simulink model "PhysicalLeanBroth"  (R2026a)
settings: Solver=VariableStepAuto  StopTime=14400
undefined symbols (not defined in the file or in its folder): Fault_T_Kettle1, Fault_T_Kettle2, Fault_T_Pack, Fault_T_Prep, Fault_T_QC, LB_PackRate_bph, LB_QCRate_bph, LB_Resupply_bph, Recipe_Block_s, Recipe_Count, Resupply_Cutoff_T, Transport_Latency_s, Transport_Rate_bph
settings Model: DataDictionary=PhysicalLeanBrothData.sldd  Creator=sarah  LastModifiedBy=sarah

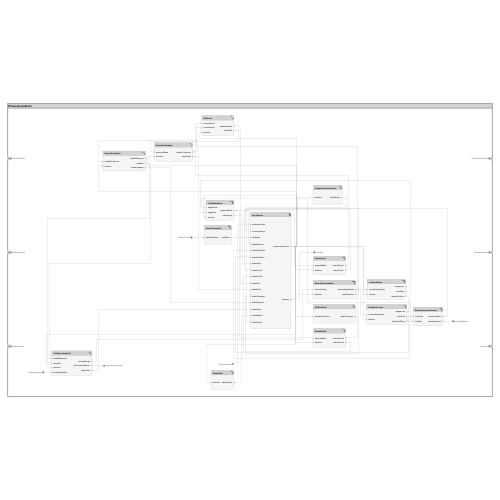
[thumbnail: Simulink's stored preview of the top-level diagram]
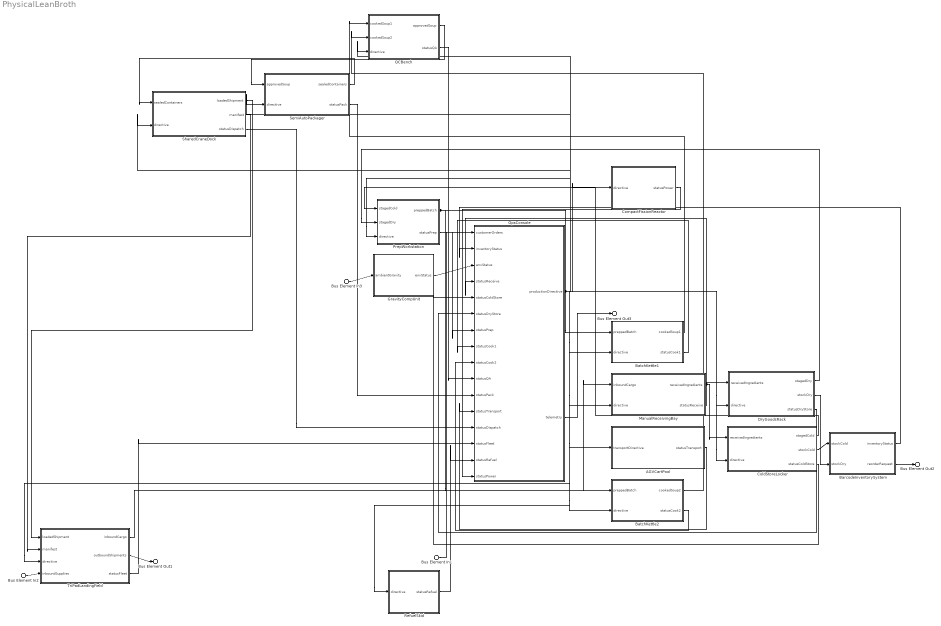
== system PhysicalLeanBroth ==
  Bus Element In1 : Inport  PortName=CustomerOrders
  Bus Element In2 : Inport  Port=2  PortName=InboundSupplies
  Bus Element In3 : Inport  Port=3  PortName=AmbientGravity
  AGVCartPool : Subsystem
      settings: PortSchema="{\"entries\":[{\"content\":{\"headerSize\":26,\"margin\":15,\"minimumSpacing\":25,\"sides\":[{\"content\":{\"connectorIds\":[\"In1\"]},\"type\":\"ConnectorPlacement.EquallySpacedRectSide\",\"uuid\":\"f830f98a-8e8b-4468-adf4-d6eab644987f\"},{\"content\":{\"connectorIds\":[\"Out1\"],\"side\":\"RIGHT\"},\"type\":\"ConnectorPlacement.EquallySpacedRectSide\",\"uuid\":\"7e0d0116-b3ba-4668-b638-30d0f54ba087\"},{\"content\":{\"side\":\"TOP\"},\"type\":\"ConnectorPlacement.EquallySpacedRectSide\",\"uuid\":\"7b4146d3-46d2-45ca-8c34-b106f0d8cedd\"}]},\"type\":\"ConnectorPlacement.EquallySpacedConnector\",\"uuid\":\"3d911b2d-a78f-42ea-b869-5e09982d9f54\"}],\"packageUris\":[\"http://schema.mathworks.com/mf0/Connector/R2020b\"],\"version\":\"1.0\"}"
  BarcodeInventorySystem : Subsystem
      settings: PortSchema="{\"entries\":[{\"content\":{\"headerSize\":26,\"margin\":15,\"minimumSpacing\":25,\"sides\":[{\"content\":{\"connectorIds\":[\"In1\",\"In2\"]},\"type\":\"ConnectorPlacement.EquallySpacedRectSide\",\"uuid\":\"f830f98a-8e8b-4468-adf4-d6eab644987f\"},{\"content\":{\"connectorIds\":[\"Out1\",\"Out2\"],\"side\":\"RIGHT\"},\"type\":\"ConnectorPlacement.EquallySpacedRectSide\",\"uuid\":\"7e0d0116-b3ba-4668-b638-30d0f54ba087\"},{\"content\":{\"side\":\"TOP\"},\"type\":\"ConnectorPlacement.EquallySpacedRectSide\",\"uuid\":\"7b4146d3-46d2-45ca-8c34-b106f0d8cedd\"}]},\"type\":\"ConnectorPlacement.EquallySpacedConnector\",\"uuid\":\"3d911b2d-a78f-42ea-b869-5e09982d9f54\"}],\"packageUris\":[\"http://schema.mathworks.com/mf0/Connector/R2020b\"],\"version\":\"1.0\"}"
  BatchKettle1 : Subsystem
      settings: PortSchema="{\"entries\":[{\"content\":{\"headerSize\":26,\"margin\":15,\"minimumSpacing\":25,\"sides\":[{\"content\":{\"connectorIds\":[\"In1\",\"In2\"]},\"type\":\"ConnectorPlacement.EquallySpacedRectSide\",\"uuid\":\"f830f98a-8e8b-4468-adf4-d6eab644987f\"},{\"content\":{\"connectorIds\":[\"Out1\",\"Out2\"],\"side\":\"RIGHT\"},\"type\":\"ConnectorPlacement.EquallySpacedRectSide\",\"uuid\":\"7e0d0116-b3ba-4668-b638-30d0f54ba087\"},{\"content\":{\"side\":\"TOP\"},\"type\":\"ConnectorPlacement.EquallySpacedRectSide\",\"uuid\":\"7b4146d3-46d2-45ca-8c34-b106f0d8cedd\"}]},\"type\":\"ConnectorPlacement.EquallySpacedConnector\",\"uuid\":\"3d911b2d-a78f-42ea-b869-5e09982d9f54\"}],\"packageUris\":[\"http://schema.mathworks.com/mf0/Connector/R2020b\"],\"version\":\"1.0\"}"
  BatchKettle2 : Subsystem
      settings: PortSchema="{\"entries\":[{\"content\":{\"headerSize\":26,\"margin\":15,\"minimumSpacing\":25,\"sides\":[{\"content\":{\"connectorIds\":[\"In1\",\"In2\"]},\"type\":\"ConnectorPlacement.EquallySpacedRectSide\",\"uuid\":\"f830f98a-8e8b-4468-adf4-d6eab644987f\"},{\"content\":{\"connectorIds\":[\"Out1\",\"Out2\"],\"side\":\"RIGHT\"},\"type\":\"ConnectorPlacement.EquallySpacedRectSide\",\"uuid\":\"7e0d0116-b3ba-4668-b638-30d0f54ba087\"},{\"content\":{\"side\":\"TOP\"},\"type\":\"ConnectorPlacement.EquallySpacedRectSide\",\"uuid\":\"7b4146d3-46d2-45ca-8c34-b106f0d8cedd\"}]},\"type\":\"ConnectorPlacement.EquallySpacedConnector\",\"uuid\":\"3d911b2d-a78f-42ea-b869-5e09982d9f54\"}],\"packageUris\":[\"http://schema.mathworks.com/mf0/Connector/R2020b\"],\"version\":\"1.0\"}"
  ColdStoreLocker : Subsystem
      settings: PortSchema="{\"entries\":[{\"content\":{\"headerSize\":26,\"margin\":15,\"minimumSpacing\":25,\"sides\":[{\"content\":{\"connectorIds\":[\"In1\",\"In2\"]},\"type\":\"ConnectorPlacement.EquallySpacedRectSide\",\"uuid\":\"f830f98a-8e8b-4468-adf4-d6eab644987f\"},{\"content\":{\"connectorIds\":[\"Out1\",\"Out2\",\"Out3\"],\"side\":\"RIGHT\"},\"type\":\"ConnectorPlacement.EquallySpacedRectSide\",\"uuid\":\"7e0d0116-b3ba-4668-b638-30d0f54ba087\"},{\"content\":{\"side\":\"TOP\"},\"type\":\"ConnectorPlacement.EquallySpacedRectSide\",\"uuid\":\"7b4146d3-46d2-45ca-8c34-b106f0d8cedd\"}]},\"type\":\"ConnectorPlacement.EquallySpacedConnector\",\"uuid\":\"3d911b2d-a78f-42ea-b869-5e09982d9f54\"}],\"packageUris\":[\"http://schema.mathworks.com/mf0/Connector/R2020b\"],\"version\":\"1.0\"}"
  CompactFissionReactor : Subsystem
      settings: PortSchema="{\"entries\":[{\"content\":{\"headerSize\":26,\"margin\":15,\"minimumSpacing\":25,\"sides\":[{\"content\":{\"connectorIds\":[\"In1\"]},\"type\":\"ConnectorPlacement.EquallySpacedRectSide\",\"uuid\":\"f830f98a-8e8b-4468-adf4-d6eab644987f\"},{\"content\":{\"connectorIds\":[\"Out1\"],\"side\":\"RIGHT\"},\"type\":\"ConnectorPlacement.EquallySpacedRectSide\",\"uuid\":\"7e0d0116-b3ba-4668-b638-30d0f54ba087\"},{\"content\":{\"side\":\"TOP\"},\"type\":\"ConnectorPlacement.EquallySpacedRectSide\",\"uuid\":\"7b4146d3-46d2-45ca-8c34-b106f0d8cedd\"}]},\"type\":\"ConnectorPlacement.EquallySpacedConnector\",\"uuid\":\"3d911b2d-a78f-42ea-b869-5e09982d9f54\"}],\"packageUris\":[\"http://schema.mathworks.com/mf0/Connector/R2020b\"],\"version\":\"1.0\"}"
  DryGoodsRack : Subsystem
      settings: PortSchema="{\"entries\":[{\"content\":{\"headerSize\":26,\"margin\":15,\"minimumSpacing\":25,\"sides\":[{\"content\":{\"connectorIds\":[\"In1\",\"In2\"]},\"type\":\"ConnectorPlacement.EquallySpacedRectSide\",\"uuid\":\"f830f98a-8e8b-4468-adf4-d6eab644987f\"},{\"content\":{\"connectorIds\":[\"Out1\",\"Out2\",\"Out3\"],\"side\":\"RIGHT\"},\"type\":\"ConnectorPlacement.EquallySpacedRectSide\",\"uuid\":\"7e0d0116-b3ba-4668-b638-30d0f54ba087\"},{\"content\":{\"side\":\"TOP\"},\"type\":\"ConnectorPlacement.EquallySpacedRectSide\",\"uuid\":\"7b4146d3-46d2-45ca-8c34-b106f0d8cedd\"}]},\"type\":\"ConnectorPlacement.EquallySpacedConnector\",\"uuid\":\"3d911b2d-a78f-42ea-b869-5e09982d9f54\"}],\"packageUris\":[\"http://schema.mathworks.com/mf0/Connector/R2020b\"],\"version\":\"1.0\"}"
  GravityCompUnit : Subsystem
      settings: PortSchema="{\"entries\":[{\"content\":{\"headerSize\":26,\"margin\":15,\"minimumSpacing\":25,\"sides\":[{\"content\":{\"connectorIds\":[\"In1\"]},\"type\":\"ConnectorPlacement.EquallySpacedRectSide\",\"uuid\":\"f830f98a-8e8b-4468-adf4-d6eab644987f\"},{\"content\":{\"connectorIds\":[\"Out1\"],\"side\":\"RIGHT\"},\"type\":\"ConnectorPlacement.EquallySpacedRectSide\",\"uuid\":\"7e0d0116-b3ba-4668-b638-30d0f54ba087\"},{\"content\":{\"side\":\"TOP\"},\"type\":\"ConnectorPlacement.EquallySpacedRectSide\",\"uuid\":\"7b4146d3-46d2-45ca-8c34-b106f0d8cedd\"}]},\"type\":\"ConnectorPlacement.EquallySpacedConnector\",\"uuid\":\"3d911b2d-a78f-42ea-b869-5e09982d9f54\"}],\"packageUris\":[\"http://schema.mathworks.com/mf0/Connector/R2020b\"],\"version\":\"1.0\"}"
  ManualReceivingBay : Subsystem
      settings: PortSchema="{\"entries\":[{\"content\":{\"headerSize\":26,\"margin\":15,\"minimumSpacing\":25,\"sides\":[{\"content\":{\"connectorIds\":[\"In1\",\"In2\"]},\"type\":\"ConnectorPlacement.EquallySpacedRectSide\",\"uuid\":\"f830f98a-8e8b-4468-adf4-d6eab644987f\"},{\"content\":{\"connectorIds\":[\"Out1\",\"Out2\"],\"side\":\"RIGHT\"},\"type\":\"ConnectorPlacement.EquallySpacedRectSide\",\"uuid\":\"7e0d0116-b3ba-4668-b638-30d0f54ba087\"},{\"content\":{\"side\":\"TOP\"},\"type\":\"ConnectorPlacement.EquallySpacedRectSide\",\"uuid\":\"7b4146d3-46d2-45ca-8c34-b106f0d8cedd\"}]},\"type\":\"ConnectorPlacement.EquallySpacedConnector\",\"uuid\":\"3d911b2d-a78f-42ea-b869-5e09982d9f54\"}],\"packageUris\":[\"http://schema.mathworks.com/mf0/Connector/R2020b\"],\"version\":\"1.0\"}"
  OpsConsole : Subsystem
      settings: PortSchema="{\"entries\":[{\"content\":{\"headerSize\":26,\"margin\":15,\"minimumSpacing\":25,\"sides\":[{\"content\":{\"connectorIds\":[\"In1\",\"In2\",\"In3\",\"In4\",\"In5\",\"In6\",\"In7\",\"In8\",\"In9\",\"In10\",\"In11\",\"In12\",\"In13\",\"In14\",\"In15\",\"In16\"]},\"type\":\"ConnectorPlacement.EquallySpacedRectSide\",\"uuid\":\"f830f98a-8e8b-4468-adf4-d6eab644987f\"},{\"content\":{\"connectorIds\":[\"Out1\",\"Out2\"],\"side\":\"RIGHT\"},\"type\":\"ConnectorPlacement.EquallySpacedRectSide\",\"uuid\":\"7e0d0116-b3ba-4668-b638-30d0f54ba087\"},{\"content\":{\"side\":\"TOP\"},\"type\":\"ConnectorPlacement.EquallySpacedRectSide\",\"uuid\":\"7b4146d3-46d2-45ca-8c34-b106f0d8cedd\"}]},\"type\":\"ConnectorPlacement.EquallySpacedConnector\",\"uuid\":\"3d911b2d-a78f-42ea-b869-5e09982d9f54\"}],\"packageUris\":[\"http://schema.mathworks.com/mf0/Connector/R2020b\"],\"version\":\"1.0\"}"
  PrepWorkstation : Subsystem
      settings: PortSchema="{\"entries\":[{\"content\":{\"headerSize\":26,\"margin\":15,\"minimumSpacing\":25,\"sides\":[{\"content\":{\"connectorIds\":[\"In1\",\"In2\",\"In3\"]},\"type\":\"ConnectorPlacement.EquallySpacedRectSide\",\"uuid\":\"f830f98a-8e8b-4468-adf4-d6eab644987f\"},{\"content\":{\"connectorIds\":[\"Out1\",\"Out2\"],\"side\":\"RIGHT\"},\"type\":\"ConnectorPlacement.EquallySpacedRectSide\",\"uuid\":\"7e0d0116-b3ba-4668-b638-30d0f54ba087\"},{\"content\":{\"side\":\"TOP\"},\"type\":\"ConnectorPlacement.EquallySpacedRectSide\",\"uuid\":\"7b4146d3-46d2-45ca-8c34-b106f0d8cedd\"}]},\"type\":\"ConnectorPlacement.EquallySpacedConnector\",\"uuid\":\"3d911b2d-a78f-42ea-b869-5e09982d9f54\"}],\"packageUris\":[\"http://schema.mathworks.com/mf0/Connector/R2020b\"],\"version\":\"1.0\"}"
  QCBench : Subsystem
      settings: PortSchema="{\"entries\":[{\"content\":{\"headerSize\":26,\"margin\":15,\"minimumSpacing\":25,\"sides\":[{\"content\":{\"connectorIds\":[\"In1\",\"In2\",\"In3\"]},\"type\":\"ConnectorPlacement.EquallySpacedRectSide\",\"uuid\":\"f830f98a-8e8b-4468-adf4-d6eab644987f\"},{\"content\":{\"connectorIds\":[\"Out1\",\"Out2\"],\"side\":\"RIGHT\"},\"type\":\"ConnectorPlacement.EquallySpacedRectSide\",\"uuid\":\"7e0d0116-b3ba-4668-b638-30d0f54ba087\"},{\"content\":{\"side\":\"TOP\"},\"type\":\"ConnectorPlacement.EquallySpacedRectSide\",\"uuid\":\"7b4146d3-46d2-45ca-8c34-b106f0d8cedd\"}]},\"type\":\"ConnectorPlacement.EquallySpacedConnector\",\"uuid\":\"3d911b2d-a78f-42ea-b869-5e09982d9f54\"}],\"packageUris\":[\"http://schema.mathworks.com/mf0/Connector/R2020b\"],\"version\":\"1.0\"}"
  RefuelSkid : Subsystem
      settings: PortSchema="{\"entries\":[{\"content\":{\"headerSize\":26,\"margin\":15,\"minimumSpacing\":25,\"sides\":[{\"content\":{\"connectorIds\":[\"In1\"]},\"type\":\"ConnectorPlacement.EquallySpacedRectSide\",\"uuid\":\"f830f98a-8e8b-4468-adf4-d6eab644987f\"},{\"content\":{\"connectorIds\":[\"Out1\"],\"side\":\"RIGHT\"},\"type\":\"ConnectorPlacement.EquallySpacedRectSide\",\"uuid\":\"7e0d0116-b3ba-4668-b638-30d0f54ba087\"},{\"content\":{\"side\":\"TOP\"},\"type\":\"ConnectorPlacement.EquallySpacedRectSide\",\"uuid\":\"7b4146d3-46d2-45ca-8c34-b106f0d8cedd\"}]},\"type\":\"ConnectorPlacement.EquallySpacedConnector\",\"uuid\":\"3d911b2d-a78f-42ea-b869-5e09982d9f54\"}],\"packageUris\":[\"http://schema.mathworks.com/mf0/Connector/R2020b\"],\"version\":\"1.0\"}"
  SemiAutoPackager : Subsystem
      settings: PortSchema="{\"entries\":[{\"content\":{\"headerSize\":26,\"margin\":15,\"minimumSpacing\":25,\"sides\":[{\"content\":{\"connectorIds\":[\"In1\",\"In2\"]},\"type\":\"ConnectorPlacement.EquallySpacedRectSide\",\"uuid\":\"f830f98a-8e8b-4468-adf4-d6eab644987f\"},{\"content\":{\"connectorIds\":[\"Out1\",\"Out2\"],\"side\":\"RIGHT\"},\"type\":\"ConnectorPlacement.EquallySpacedRectSide\",\"uuid\":\"7e0d0116-b3ba-4668-b638-30d0f54ba087\"},{\"content\":{\"side\":\"TOP\"},\"type\":\"ConnectorPlacement.EquallySpacedRectSide\",\"uuid\":\"7b4146d3-46d2-45ca-8c34-b106f0d8cedd\"}]},\"type\":\"ConnectorPlacement.EquallySpacedConnector\",\"uuid\":\"3d911b2d-a78f-42ea-b869-5e09982d9f54\"}],\"packageUris\":[\"http://schema.mathworks.com/mf0/Connector/R2020b\"],\"version\":\"1.0\"}"
  SharedCraneDock : Subsystem
      settings: PortSchema="{\"entries\":[{\"content\":{\"headerSize\":26,\"margin\":15,\"minimumSpacing\":25,\"sides\":[{\"content\":{\"connectorIds\":[\"In1\",\"In2\"]},\"type\":\"ConnectorPlacement.EquallySpacedRectSide\",\"uuid\":\"f830f98a-8e8b-4468-adf4-d6eab644987f\"},{\"content\":{\"connectorIds\":[\"Out1\",\"Out2\",\"Out3\"],\"side\":\"RIGHT\"},\"type\":\"ConnectorPlacement.EquallySpacedRectSide\",\"uuid\":\"7e0d0116-b3ba-4668-b638-30d0f54ba087\"},{\"content\":{\"side\":\"TOP\"},\"type\":\"ConnectorPlacement.EquallySpacedRectSide\",\"uuid\":\"7b4146d3-46d2-45ca-8c34-b106f0d8cedd\"}]},\"type\":\"ConnectorPlacement.EquallySpacedConnector\",\"uuid\":\"3d911b2d-a78f-42ea-b869-5e09982d9f54\"}],\"packageUris\":[\"http://schema.mathworks.com/mf0/Connector/R2020b\"],\"version\":\"1.0\"}"
  TriPadLandingField : Subsystem
      settings: PortSchema="{\"entries\":[{\"content\":{\"headerSize\":26,\"margin\":15,\"minimumSpacing\":25,\"sides\":[{\"content\":{\"connectorIds\":[\"In1\",\"In2\",\"In3\",\"In4\"]},\"type\":\"ConnectorPlacement.EquallySpacedRectSide\",\"uuid\":\"f830f98a-8e8b-4468-adf4-d6eab644987f\"},{\"content\":{\"connectorIds\":[\"Out1\",\"Out2\",\"Out3\"],\"side\":\"RIGHT\"},\"type\":\"ConnectorPlacement.EquallySpacedRectSide\",\"uuid\":\"7e0d0116-b3ba-4668-b638-30d0f54ba087\"},{\"content\":{\"side\":\"TOP\"},\"type\":\"ConnectorPlacement.EquallySpacedRectSide\",\"uuid\":\"7b4146d3-46d2-45ca-8c34-b106f0d8cedd\"}]},\"type\":\"ConnectorPlacement.EquallySpacedConnector\",\"uuid\":\"3d911b2d-a78f-42ea-b869-5e09982d9f54\"}],\"packageUris\":[\"http://schema.mathworks.com/mf0/Connector/R2020b\"],\"version\":\"1.0\"}"
  Bus Element Out1 : Outport  PortName=OutboundShipments
  Bus Element Out2 : Outport  Port=2  PortName=ReorderRequests
  Bus Element Out3 : Outport  Port=3  PortName=Telemetry
  wires:
  GravityCompUnit/1(envStatus) -> OpsConsole/3(envStatus)
  Bus Element In2/1 -> TriPadLandingField/4(inboundSupplies)
  BatchKettle2/1(cookedSoup2) -> QCBench/2(cookedSoup2)
  ManualReceivingBay/2(statusReceive) -> OpsConsole/4(statusReceive)
  TriPadLandingField/1(inboundCargo) -> ManualReceivingBay/1(inboundCargo)
  TriPadLandingField/2(outboundShipments) -> Bus Element Out1/1
  SemiAutoPackager/1(sealedContainers) -> SharedCraneDock/1(sealedContainers)
  TriPadLandingField/3(statusFleet) -> OpsConsole/14(statusFleet)
  SharedCraneDock/1(loadedShipment) -> TriPadLandingField/1(loadedShipment)
  SharedCraneDock/2(manifest) -> TriPadLandingField/2(manifest)
  SharedCraneDock/3(statusDispatch) -> OpsConsole/13(statusDispatch)
  BarcodeInventorySystem/2(reorderRequest) -> Bus Element Out2/1
  CompactFissionReactor/1(statusPower) -> OpsConsole/16(statusPower)
  SemiAutoPackager/2(statusPack) -> OpsConsole/11(statusPack)
  QCBench/1(approvedSoup) -> SemiAutoPackager/1(approvedSoup)
  Bus Element In3/1 -> GravityCompUnit/1(ambientGravity)
  QCBench/2(statusQA) -> OpsConsole/10(statusQA)
  PrepWorkstation/1(preppedBatch) -> BatchKettle1/1(preppedBatch), BatchKettle2/1(preppedBatch)
  OpsConsole/1(productionDirective) -> QCBench/3(directive), SemiAutoPackager/2(directive), SharedCraneDock/2(directive), TriPadLandingField/3(directive), RefuelSkid/1(directive), ColdStoreLocker/2(directive), AGVCartPool/1(transportDirective), ManualReceivingBay/2(directive), DryGoodsRack/2(directive), BatchKettle1/2(directive), CompactFissionReactor/1(directive), BatchKettle2/2(directive), PrepWorkstation/3(directive)
  PrepWorkstation/2(statusPrep) -> OpsConsole/7(statusPrep)
  Bus Element In1/1 -> OpsConsole/1(customerOrders)
  RefuelSkid/1(statusRefuel) -> OpsConsole/15(statusRefuel)
  OpsConsole/2(telemetry) -> Bus Element Out3/1
  BatchKettle1/1(cookedSoup1) -> QCBench/1(cookedSoup1)
  BatchKettle1/2(statusCook1) -> OpsConsole/8(statusCook1)
  ManualReceivingBay/1(receivedIngredients) -> DryGoodsRack/1(receivedIngredients), ColdStoreLocker/1(receivedIngredients)
  AGVCartPool/1(statusTransport) -> OpsConsole/12(statusTransport)
  BatchKettle2/2(statusCook2) -> OpsConsole/9(statusCook2)
  ColdStoreLocker/1(stagedCold) -> PrepWorkstation/1(stagedCold)
  DryGoodsRack/1(stagedDry) -> PrepWorkstation/2(stagedDry)
  ColdStoreLocker/2(stockCold) -> BarcodeInventorySystem/1(stockCold)
  DryGoodsRack/2(stockDry) -> BarcodeInventorySystem/2(stockDry)
  BarcodeInventorySystem/1(inventoryStatus) -> OpsConsole/2(inventoryStatus)
  DryGoodsRack/3(statusDryStore) -> OpsConsole/6(statusDryStore)
  ColdStoreLocker/3(statusColdStore) -> OpsConsole/5(statusColdStore)

== system PhysicalLeanBroth/AGVCartPool ==
  in_transportDirective : Inport  PortName=transportDirective
  statusTransport_c1 : Constant
  statusTransport_c2 : Constant
  statusTransport_c3 : Constant  Value=0
  statusTransport_c4 : Constant  Value=8
  statusTransport_h : Constant
  out_statusTransport : Outport  PortName=statusTransport  Element=unitId
  statusTransport_el2 : Outport  PortName=statusTransport  Element=opState
  statusTransport_el3 : Outport  PortName=statusTransport  Element=faultCode
  statusTransport_el4 : Outport  PortName=statusTransport  Element=power_kW
  statusTransport_el5 : Outport  PortName=statusTransport  Element=health
  wires:
  statusTransport_h/1 -> statusTransport_el5/1
  statusTransport_c1/1 -> out_statusTransport/1
  statusTransport_c2/1 -> statusTransport_el2/1
  statusTransport_c3/1 -> statusTransport_el3/1
  statusTransport_c4/1 -> statusTransport_el4/1

== system PhysicalLeanBroth/BarcodeInventorySystem ==
  in_stockCold : Inport  PortName=stockCold
  in_stockDry : Inport  Port=2  PortName=stockDry
  inventoryStatus_c1 : Constant
  inventoryStatus_c2 : Constant  Value=500
  inventoryStatus_c3 : Constant  Value=0
  reorderRequest_c1 : Constant
  reorderRequest_c2 : Constant  Value=0
  reorderRequest_c3 : Constant  Value=0
  out_inventoryStatus : Outport  PortName=inventoryStatus  Element=itemId
  inventoryStatus_el2 : Outport  PortName=inventoryStatus  Element=qty_units
  inventoryStatus_el3 : Outport  PortName=inventoryStatus  Element=error_pct
  out_reorderRequest : Outport  Port=2  PortName=reorderRequest  Element=itemId
  reorderRequest_el2 : Outport  Port=2  PortName=reorderRequest  Element=qty_units
  reorderRequest_el3 : Outport  Port=2  PortName=reorderRequest  Element=error_pct
  wires:
  reorderRequest_c2/1 -> reorderRequest_el2/1
  reorderRequest_c3/1 -> reorderRequest_el3/1
  reorderRequest_c1/1 -> out_reorderRequest/1
  inventoryStatus_c1/1 -> out_inventoryStatus/1
  inventoryStatus_c3/1 -> inventoryStatus_el3/1
  inventoryStatus_c2/1 -> inventoryStatus_el2/1

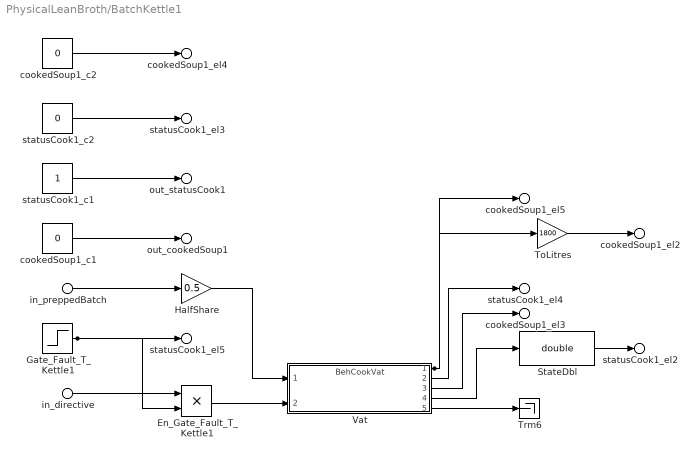
== system PhysicalLeanBroth/BatchKettle1 ==
  in_preppedBatch : Inport  PortName=preppedBatch  Element=flow_bps
  in_directive : Inport  Port=2  PortName=directive  Element=setpoint
  En_Gate_Fault_T_Kettle1 : Product
  Gate_Fault_T_Kettle1 : Step  Time=Fault_T_Kettle1  InitialValue=1  FinalValue=0  SampleTime=0
  HalfShare : Gain  Gain=0.5
  StateDbl : DataTypeConversion  OutDataTypeStr=double  SaturateOnIntegerOverflow=off  RndMeth=Floor
  ToLitres : Gain  Gain=1800
  Trm6 : Terminator
  Vat : ModelReference  ModelNameDialog=BehCookVat  UsingDefaultArgumentValue=0,0,0,0,0,0,0,0  SimulationMode=Normal  ModelReferenceVersion=1.8
  cookedSoup1_c1 : Constant  Value=0
  cookedSoup1_c2 : Constant  Value=0
  statusCook1_c1 : Constant
  statusCook1_c2 : Constant  Value=0
  out_cookedSoup1 : Outport  PortName=cookedSoup1  Element=batchId
  cookedSoup1_el2 : Outport  PortName=cookedSoup1  Element=volume_L
  cookedSoup1_el3 : Outport  PortName=cookedSoup1  Element=temp_C
  cookedSoup1_el4 : Outport  PortName=cookedSoup1  Element=contamination_ppm
  cookedSoup1_el5 : Outport  PortName=cookedSoup1  Element=flow_bps
  out_statusCook1 : Outport  Port=2  PortName=statusCook1  Element=unitId
  statusCook1_el2 : Outport  Port=2  PortName=statusCook1  Element=opState
  statusCook1_el3 : Outport  Port=2  PortName=statusCook1  Element=faultCode
  statusCook1_el4 : Outport  Port=2  PortName=statusCook1  Element=power_kW
  statusCook1_el5 : Outport  Port=2  PortName=statusCook1  Element=health
  wires:
  HalfShare/1 -> Vat/1
  cookedSoup1_c2/1 -> cookedSoup1_el4/1
  statusCook1_c2/1 -> statusCook1_el3/1
  Gate_Fault_T_Kettle1/1 -> En_Gate_Fault_T_Kettle1/2, statusCook1_el5/1
  statusCook1_c1/1 -> out_statusCook1/1
  Vat/1 -> cookedSoup1_el5/1, ToLitres/1
  in_preppedBatch/1 -> HalfShare/1
  cookedSoup1_c1/1 -> out_cookedSoup1/1
  in_directive/1 -> En_Gate_Fault_T_Kettle1/1
  En_Gate_Fault_T_Kettle1/1 -> Vat/2
  Vat/2 -> statusCook1_el4/1
  Vat/3 -> cookedSoup1_el3/1
  Vat/4 -> StateDbl/1
  Vat/5 -> Trm6/1
  ToLitres/1 -> cookedSoup1_el2/1
  StateDbl/1 -> statusCook1_el2/1

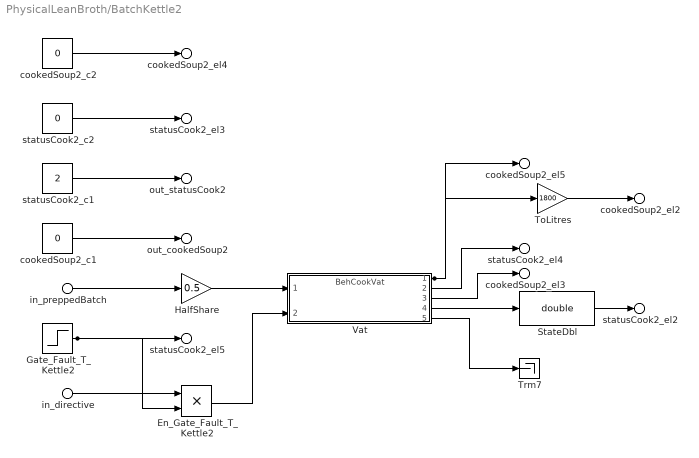
== system PhysicalLeanBroth/BatchKettle2 ==
  in_preppedBatch : Inport  PortName=preppedBatch  Element=flow_bps
  in_directive : Inport  Port=2  PortName=directive  Element=setpoint
  En_Gate_Fault_T_Kettle2 : Product
  Gate_Fault_T_Kettle2 : Step  Time=Fault_T_Kettle2  InitialValue=1  FinalValue=0  SampleTime=0
  HalfShare : Gain  Gain=0.5
  StateDbl : DataTypeConversion  OutDataTypeStr=double  SaturateOnIntegerOverflow=off  RndMeth=Floor
  ToLitres : Gain  Gain=1800
  Trm7 : Terminator
  Vat : ModelReference  ModelNameDialog=BehCookVat  UsingDefaultArgumentValue=0,0,0,0,0,0,0,0  SimulationMode=Normal  ModelReferenceVersion=1.8
  cookedSoup2_c1 : Constant  Value=0
  cookedSoup2_c2 : Constant  Value=0
  statusCook2_c1 : Constant  Value=2
  statusCook2_c2 : Constant  Value=0
  out_cookedSoup2 : Outport  PortName=cookedSoup2  Element=batchId
  cookedSoup2_el2 : Outport  PortName=cookedSoup2  Element=volume_L
  cookedSoup2_el3 : Outport  PortName=cookedSoup2  Element=temp_C
  cookedSoup2_el4 : Outport  PortName=cookedSoup2  Element=contamination_ppm
  cookedSoup2_el5 : Outport  PortName=cookedSoup2  Element=flow_bps
  out_statusCook2 : Outport  Port=2  PortName=statusCook2  Element=unitId
  statusCook2_el2 : Outport  Port=2  PortName=statusCook2  Element=opState
  statusCook2_el3 : Outport  Port=2  PortName=statusCook2  Element=faultCode
  statusCook2_el4 : Outport  Port=2  PortName=statusCook2  Element=power_kW
  statusCook2_el5 : Outport  Port=2  PortName=statusCook2  Element=health
  wires:
  cookedSoup2_c2/1 -> cookedSoup2_el4/1
  in_directive/1 -> En_Gate_Fault_T_Kettle2/1
  Gate_Fault_T_Kettle2/1 -> En_Gate_Fault_T_Kettle2/2, statusCook2_el5/1
  statusCook2_c2/1 -> statusCook2_el3/1
  cookedSoup2_c1/1 -> out_cookedSoup2/1
  statusCook2_c1/1 -> out_statusCook2/1
  in_preppedBatch/1 -> HalfShare/1
  HalfShare/1 -> Vat/1
  En_Gate_Fault_T_Kettle2/1 -> Vat/2
  Vat/1 -> cookedSoup2_el5/1, ToLitres/1
  Vat/2 -> statusCook2_el4/1
  Vat/3 -> cookedSoup2_el3/1
  Vat/4 -> StateDbl/1
  Vat/5 -> Trm7/1
  ToLitres/1 -> cookedSoup2_el2/1
  StateDbl/1 -> statusCook2_el2/1

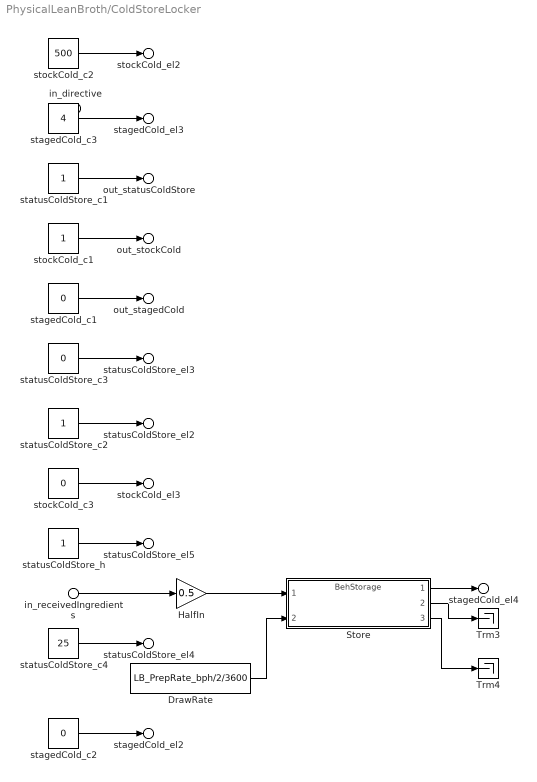
== system PhysicalLeanBroth/ColdStoreLocker ==
  in_receivedIngredients : Inport  PortName=receivedIngredients  Element=flow_bps
  in_directive : Inport  Port=2  PortName=directive  Element=setpoint
  DrawRate : Constant  Value=LB_PrepRate_bph/2/3600
  HalfIn : Gain  Gain=0.5
  Store : ModelReference  ModelNameDialog=BehStorage  UsingDefaultArgumentValue=0,0  SimulationMode=Normal  ModelReferenceVersion=1.3
  Trm3 : Terminator
  Trm4 : Terminator
  stagedCold_c1 : Constant  Value=0
  stagedCold_c2 : Constant  Value=0
  stagedCold_c3 : Constant  Value=4
  statusColdStore_c1 : Constant
  statusColdStore_c2 : Constant
  statusColdStore_c3 : Constant  Value=0
  statusColdStore_c4 : Constant  Value=25
  statusColdStore_h : Constant
  stockCold_c1 : Constant
  stockCold_c2 : Constant  Value=500
  stockCold_c3 : Constant  Value=0
  out_stagedCold : Outport  PortName=stagedCold  Element=palletId
  stagedCold_el2 : Outport  PortName=stagedCold  Element=mass_kg
  stagedCold_el3 : Outport  PortName=stagedCold  Element=temp_C
  stagedCold_el4 : Outport  PortName=stagedCold  Element=flow_bps
  out_stockCold : Outport  Port=2  PortName=stockCold  Element=itemId
  stockCold_el2 : Outport  Port=2  PortName=stockCold  Element=qty_units
  stockCold_el3 : Outport  Port=2  PortName=stockCold  Element=error_pct
  out_statusColdStore : Outport  Port=3  PortName=statusColdStore  Element=unitId
  statusColdStore_el2 : Outport  Port=3  PortName=statusColdStore  Element=opState
  statusColdStore_el3 : Outport  Port=3  PortName=statusColdStore  Element=faultCode
  statusColdStore_el4 : Outport  Port=3  PortName=statusColdStore  Element=power_kW
  statusColdStore_el5 : Outport  Port=3  PortName=statusColdStore  Element=health
  wires:
  stockCold_c1/1 -> out_stockCold/1
  stockCold_c3/1 -> stockCold_el3/1
  stockCold_c2/1 -> stockCold_el2/1
  Store/1 -> stagedCold_el4/1
  stagedCold_c3/1 -> stagedCold_el3/1
  statusColdStore_c1/1 -> out_statusColdStore/1
  stagedCold_c1/1 -> out_stagedCold/1
  statusColdStore_c3/1 -> statusColdStore_el3/1
  statusColdStore_c2/1 -> statusColdStore_el2/1
  statusColdStore_h/1 -> statusColdStore_el5/1
  in_receivedIngredients/1 -> HalfIn/1
  statusColdStore_c4/1 -> statusColdStore_el4/1
  stagedCold_c2/1 -> stagedCold_el2/1
  HalfIn/1 -> Store/1
  DrawRate/1 -> Store/2
  Store/2 -> Trm3/1
  Store/3 -> Trm4/1

== system PhysicalLeanBroth/CompactFissionReactor ==
  in_directive : Inport  PortName=directive
  statusPower_c1 : Constant
  statusPower_c2 : Constant
  statusPower_c3 : Constant  Value=0
  statusPower_c4 : Constant  Value=0
  statusPower_h : Constant
  out_statusPower : Outport  PortName=statusPower  Element=unitId
  statusPower_el2 : Outport  PortName=statusPower  Element=opState
  statusPower_el3 : Outport  PortName=statusPower  Element=faultCode
  statusPower_el4 : Outport  PortName=statusPower  Element=power_kW
  statusPower_el5 : Outport  PortName=statusPower  Element=health
  wires:
  statusPower_h/1 -> statusPower_el5/1
  statusPower_c1/1 -> out_statusPower/1
  statusPower_c3/1 -> statusPower_el3/1
  statusPower_c2/1 -> statusPower_el2/1
  statusPower_c4/1 -> statusPower_el4/1

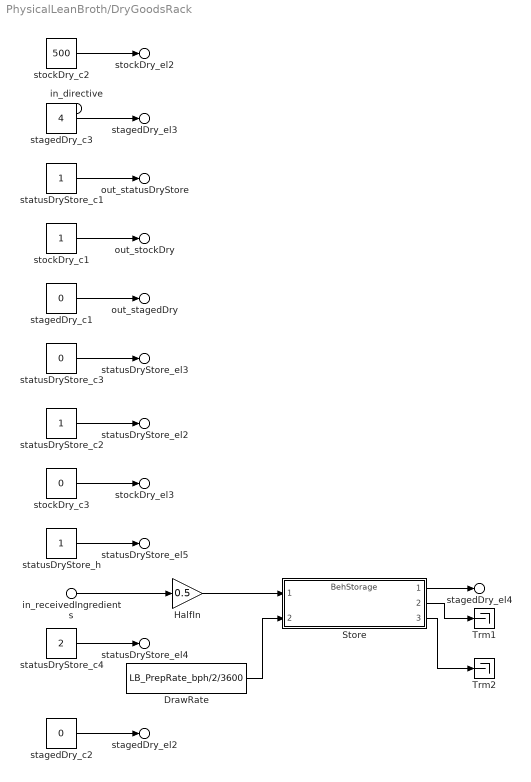
== system PhysicalLeanBroth/DryGoodsRack ==
  in_receivedIngredients : Inport  PortName=receivedIngredients  Element=flow_bps
  in_directive : Inport  Port=2  PortName=directive  Element=setpoint
  DrawRate : Constant  Value=LB_PrepRate_bph/2/3600
  HalfIn : Gain  Gain=0.5
  Store : ModelReference  ModelNameDialog=BehStorage  UsingDefaultArgumentValue=0,0  SimulationMode=Normal  ModelReferenceVersion=1.3
  Trm1 : Terminator
  Trm2 : Terminator
  stagedDry_c1 : Constant  Value=0
  stagedDry_c2 : Constant  Value=0
  stagedDry_c3 : Constant  Value=4
  statusDryStore_c1 : Constant
  statusDryStore_c2 : Constant
  statusDryStore_c3 : Constant  Value=0
  statusDryStore_c4 : Constant  Value=2
  statusDryStore_h : Constant
  stockDry_c1 : Constant
  stockDry_c2 : Constant  Value=500
  stockDry_c3 : Constant  Value=0
  out_stagedDry : Outport  PortName=stagedDry  Element=palletId
  stagedDry_el2 : Outport  PortName=stagedDry  Element=mass_kg
  stagedDry_el3 : Outport  PortName=stagedDry  Element=temp_C
  stagedDry_el4 : Outport  PortName=stagedDry  Element=flow_bps
  out_stockDry : Outport  Port=2  PortName=stockDry  Element=itemId
  stockDry_el2 : Outport  Port=2  PortName=stockDry  Element=qty_units
  stockDry_el3 : Outport  Port=2  PortName=stockDry  Element=error_pct
  out_statusDryStore : Outport  Port=3  PortName=statusDryStore  Element=unitId
  statusDryStore_el2 : Outport  Port=3  PortName=statusDryStore  Element=opState
  statusDryStore_el3 : Outport  Port=3  PortName=statusDryStore  Element=faultCode
  statusDryStore_el4 : Outport  Port=3  PortName=statusDryStore  Element=power_kW
  statusDryStore_el5 : Outport  Port=3  PortName=statusDryStore  Element=health
  wires:
  statusDryStore_c3/1 -> statusDryStore_el3/1
  stagedDry_c3/1 -> stagedDry_el3/1
  stockDry_c2/1 -> stockDry_el2/1
  stockDry_c1/1 -> out_stockDry/1
  statusDryStore_c1/1 -> out_statusDryStore/1
  stagedDry_c1/1 -> out_stagedDry/1
  statusDryStore_c2/1 -> statusDryStore_el2/1
  stockDry_c3/1 -> stockDry_el3/1
  statusDryStore_h/1 -> statusDryStore_el5/1
  Store/1 -> stagedDry_el4/1
  in_receivedIngredients/1 -> HalfIn/1
  statusDryStore_c4/1 -> statusDryStore_el4/1
  Store/3 -> Trm2/1
  stagedDry_c2/1 -> stagedDry_el2/1
  HalfIn/1 -> Store/1
  DrawRate/1 -> Store/2
  Store/2 -> Trm1/1

== system PhysicalLeanBroth/GravityCompUnit ==
  in_ambientGravity : Inport  PortName=ambientGravity  Element=gravity_g
  envStatus_c1 : Constant  Value=100
  out_envStatus : Outport  PortName=envStatus  Element=gravity_g
  envStatus_el2 : Outport  PortName=envStatus  Element=compensation_pct
  wires:
  in_ambientGravity/1 -> out_envStatus/1  "ambientGravity"
  envStatus_c1/1 -> envStatus_el2/1

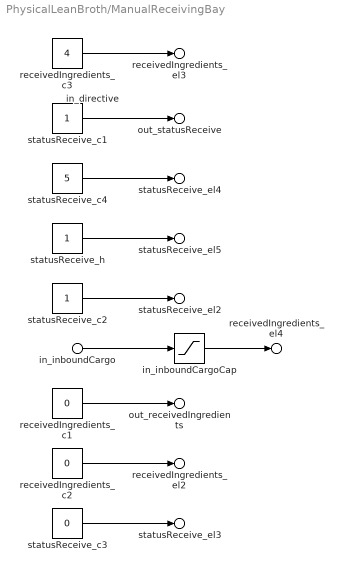
== system PhysicalLeanBroth/ManualReceivingBay ==
  in_inboundCargo : Inport  PortName=inboundCargo  Element=flow_bps
  in_directive : Inport  Port=2  PortName=directive
  in_inboundCargoCap : Saturate  UpperLimit=0.0694444444444  LowerLimit=0
  receivedIngredients_c1 : Constant  Value=0
  receivedIngredients_c2 : Constant  Value=0
  receivedIngredients_c3 : Constant  Value=4
  statusReceive_c1 : Constant
  statusReceive_c2 : Constant
  statusReceive_c3 : Constant  Value=0
  statusReceive_c4 : Constant  Value=5
  statusReceive_h : Constant
  out_receivedIngredients : Outport  PortName=receivedIngredients  Element=palletId
  receivedIngredients_el2 : Outport  PortName=receivedIngredients  Element=mass_kg
  receivedIngredients_el3 : Outport  PortName=receivedIngredients  Element=temp_C
  receivedIngredients_el4 : Outport  PortName=receivedIngredients  Element=flow_bps
  out_statusReceive : Outport  Port=2  PortName=statusReceive  Element=unitId
  statusReceive_el2 : Outport  Port=2  PortName=statusReceive  Element=opState
  statusReceive_el3 : Outport  Port=2  PortName=statusReceive  Element=faultCode
  statusReceive_el4 : Outport  Port=2  PortName=statusReceive  Element=power_kW
  statusReceive_el5 : Outport  Port=2  PortName=statusReceive  Element=health
  wires:
  receivedIngredients_c3/1 -> receivedIngredients_el3/1
  statusReceive_c1/1 -> out_statusReceive/1
  statusReceive_c4/1 -> statusReceive_el4/1
  in_inboundCargo/1 -> in_inboundCargoCap/1
  statusReceive_h/1 -> statusReceive_el5/1
  receivedIngredients_c2/1 -> receivedIngredients_el2/1
  statusReceive_c2/1 -> statusReceive_el2/1
  receivedIngredients_c1/1 -> out_receivedIngredients/1
  statusReceive_c3/1 -> statusReceive_el3/1
  in_inboundCargoCap/1 -> receivedIngredients_el4/1

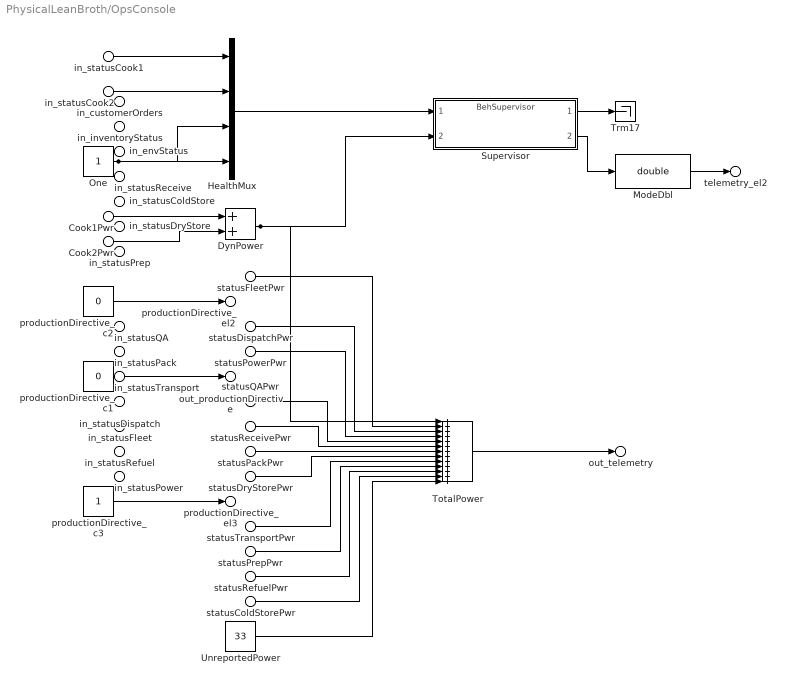
== system PhysicalLeanBroth/OpsConsole ==
  in_customerOrders : Inport  PortName=customerOrders
  in_inventoryStatus : Inport  Port=2  PortName=inventoryStatus
  in_envStatus : Inport  Port=3  PortName=envStatus
  in_statusReceive : Inport  Port=4  PortName=statusReceive
  statusReceivePwr : Inport  Port=4  PortName=statusReceive  Element=power_kW
  in_statusColdStore : Inport  Port=5  PortName=statusColdStore
  statusColdStorePwr : Inport  Port=5  PortName=statusColdStore  Element=power_kW
  in_statusDryStore : Inport  Port=6  PortName=statusDryStore
  statusDryStorePwr : Inport  Port=6  PortName=statusDryStore  Element=power_kW
  in_statusPrep : Inport  Port=7  PortName=statusPrep
  statusPrepPwr : Inport  Port=7  PortName=statusPrep  Element=power_kW
  Cook1Pwr : Inport  Port=8  PortName=statusCook1  Element=power_kW
  in_statusCook1 : Inport  Port=8  PortName=statusCook1  Element=health
  Cook2Pwr : Inport  Port=9  PortName=statusCook2  Element=power_kW
  in_statusCook2 : Inport  Port=9  PortName=statusCook2  Element=health
  in_statusQA : Inport  Port=10  PortName=statusQA
  statusQAPwr : Inport  Port=10  PortName=statusQA  Element=power_kW
  in_statusPack : Inport  Port=11  PortName=statusPack
  statusPackPwr : Inport  Port=11  PortName=statusPack  Element=power_kW
  in_statusTransport : Inport  Port=12  PortName=statusTransport
  statusTransportPwr : Inport  Port=12  PortName=statusTransport  Element=power_kW
  in_statusDispatch : Inport  Port=13  PortName=statusDispatch
  statusDispatchPwr : Inport  Port=13  PortName=statusDispatch  Element=power_kW
  in_statusFleet : Inport  Port=14  PortName=statusFleet
  statusFleetPwr : Inport  Port=14  PortName=statusFleet  Element=power_kW
  in_statusRefuel : Inport  Port=15  PortName=statusRefuel
  statusRefuelPwr : Inport  Port=15  PortName=statusRefuel  Element=power_kW
  in_statusPower : Inport  Port=16  PortName=statusPower
  statusPowerPwr : Inport  Port=16  PortName=statusPower  Element=power_kW
  DynPower : Sum
  HealthMux : Mux
  ModeDbl : DataTypeConversion  OutDataTypeStr=double  SaturateOnIntegerOverflow=off  RndMeth=Floor
  One : Constant
  Supervisor : ModelReference  ModelNameDialog=BehSupervisor  ParameterArgumentNames=NumLines  ParameterArgumentValues=LB_NumLines  UsingDefaultArgumentValue=0  SimulationMode=Normal  ModelReferenceVersion=1.6
  TotalPower : Sum  Inputs=+++++++++++++
  Trm17 : Terminator
  UnreportedPower : Constant  Value=33
  productionDirective_c1 : Constant  Value=0
  productionDirective_c2 : Constant  Value=0
  productionDirective_c3 : Constant
  out_productionDirective : Outport  PortName=productionDirective  Element=cmdType
  productionDirective_el2 : Outport  PortName=productionDirective  Element=targetId
  productionDirective_el3 : Outport  PortName=productionDirective  Element=setpoint
  out_telemetry : Outport  Port=2  PortName=telemetry  Element=totalPower_kW
  telemetry_el2 : Outport  Port=2  PortName=telemetry  Element=plantMode
  wires:
  statusColdStorePwr/1 -> TotalPower/12
  productionDirective_c2/1 -> productionDirective_el2/1
  in_statusCook1/1 -> HealthMux/1
  productionDirective_c1/1 -> out_productionDirective/1
  Supervisor/2 -> ModeDbl/1
  in_statusCook2/1 -> HealthMux/2
  statusPowerPwr/1 -> TotalPower/4
  One/1 -> HealthMux/3, HealthMux/4
  Cook1Pwr/1 -> DynPower/1
  Cook2Pwr/1 -> DynPower/2
  statusReceivePwr/1 -> TotalPower/6
  statusDispatchPwr/1 -> TotalPower/3
  productionDirective_c3/1 -> productionDirective_el3/1
  HealthMux/1 -> Supervisor/1
  DynPower/1 -> Supervisor/2, TotalPower/1
  statusFleetPwr/1 -> TotalPower/2
  statusQAPwr/1 -> TotalPower/5
  statusRefuelPwr/1 -> TotalPower/11
  statusPackPwr/1 -> TotalPower/7
  statusDryStorePwr/1 -> TotalPower/8
  statusTransportPwr/1 -> TotalPower/9
  statusPrepPwr/1 -> TotalPower/10
  UnreportedPower/1 -> TotalPower/13
  Supervisor/1 -> Trm17/1
  TotalPower/1 -> out_telemetry/1
  ModeDbl/1 -> telemetry_el2/1

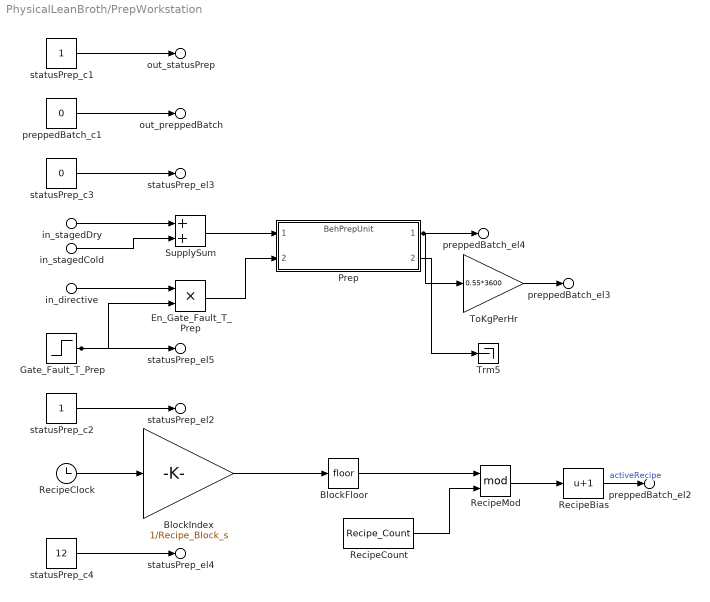
== system PhysicalLeanBroth/PrepWorkstation ==
  in_stagedCold : Inport  PortName=stagedCold  Element=flow_bps
  in_stagedDry : Inport  Port=2  PortName=stagedDry  Element=flow_bps
  in_directive : Inport  Port=3  PortName=directive  Element=setpoint
  BlockFloor : Rounding
  BlockIndex : Gain  Gain=1/Recipe_Block_s
  En_Gate_Fault_T_Prep : Product
  Gate_Fault_T_Prep : Step  Time=Fault_T_Prep  InitialValue=1  FinalValue=0  SampleTime=0
  Prep : ModelReference  ModelNameDialog=BehPrepUnit  UsingDefaultArgumentValue=0,0  SimulationMode=Normal  ModelReferenceVersion=1.4
  RecipeBias : Bias  Bias=1  SaturateOnIntegerOverflow=off
  RecipeClock : Clock
  RecipeCount : Constant  Value=Recipe_Count
  RecipeMod : Math  Operator=mod
  SupplySum : Sum
  ToKgPerHr : Gain  Gain=0.55*3600
  Trm5 : Terminator
  preppedBatch_c1 : Constant  Value=0
  statusPrep_c1 : Constant
  statusPrep_c2 : Constant
  statusPrep_c3 : Constant  Value=0
  statusPrep_c4 : Constant  Value=12
  out_preppedBatch : Outport  PortName=preppedBatch  Element=batchId
  preppedBatch_el2 : Outport  PortName=preppedBatch  Element=recipeId
  preppedBatch_el3 : Outport  PortName=preppedBatch  Element=mass_kg
  preppedBatch_el4 : Outport  PortName=preppedBatch  Element=flow_bps
  out_statusPrep : Outport  Port=2  PortName=statusPrep  Element=unitId
  statusPrep_el2 : Outport  Port=2  PortName=statusPrep  Element=opState
  statusPrep_el3 : Outport  Port=2  PortName=statusPrep  Element=faultCode
  statusPrep_el4 : Outport  Port=2  PortName=statusPrep  Element=power_kW
  statusPrep_el5 : Outport  Port=2  PortName=statusPrep  Element=health
  wires:
  Prep/1 -> preppedBatch_el4/1, ToKgPerHr/1
  in_stagedDry/1 -> SupplySum/1
  statusPrep_c1/1 -> out_statusPrep/1
  statusPrep_c3/1 -> statusPrep_el3/1
  preppedBatch_c1/1 -> out_preppedBatch/1
  RecipeClock/1 -> BlockIndex/1
  Gate_Fault_T_Prep/1 -> statusPrep_el5/1, En_Gate_Fault_T_Prep/2
  in_stagedCold/1 -> SupplySum/2
  in_directive/1 -> En_Gate_Fault_T_Prep/1
  RecipeBias/1 -> preppedBatch_el2/1  "activeRecipe"
  statusPrep_c4/1 -> statusPrep_el4/1
  statusPrep_c2/1 -> statusPrep_el2/1
  SupplySum/1 -> Prep/1
  En_Gate_Fault_T_Prep/1 -> Prep/2
  BlockIndex/1 -> BlockFloor/1
  Prep/2 -> Trm5/1
  BlockFloor/1 -> RecipeMod/1
  RecipeCount/1 -> RecipeMod/2
  ToKgPerHr/1 -> preppedBatch_el3/1
  RecipeMod/1 -> RecipeBias/1

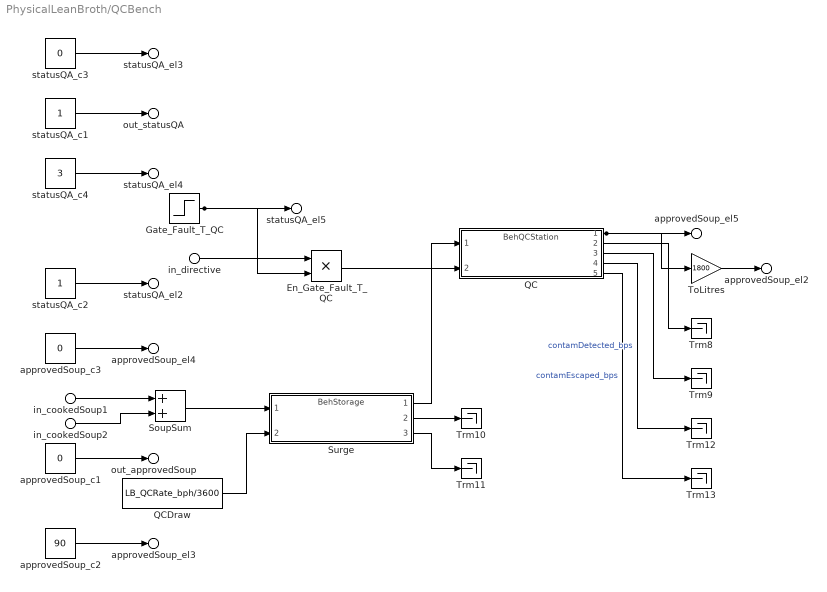
== system PhysicalLeanBroth/QCBench ==
  in_cookedSoup1 : Inport  PortName=cookedSoup1  Element=flow_bps
  in_cookedSoup2 : Inport  Port=2  PortName=cookedSoup2  Element=flow_bps
  in_directive : Inport  Port=3  PortName=directive  Element=setpoint
  En_Gate_Fault_T_QC : Product
  Gate_Fault_T_QC : Step  Time=Fault_T_QC  InitialValue=1  FinalValue=0  SampleTime=0
  QC : ModelReference  ModelNameDialog=BehQCStation  UsingDefaultArgumentValue=0,0,0,0,0,0  SimulationMode=Normal  ModelReferenceVersion=1.5
  QCDraw : Constant  Value=LB_QCRate_bph/3600
  SoupSum : Sum
  Surge : ModelReference  ModelNameDialog=BehStorage  UsingDefaultArgumentValue=0,0  SimulationMode=Normal  ModelReferenceVersion=1.3
  ToLitres : Gain  Gain=1800
  Trm{8..13} (6 alike) : Terminator
  approvedSoup_c1 : Constant  Value=0
  approvedSoup_c2 : Constant  Value=90
  approvedSoup_c3 : Constant  Value=0
  statusQA_c1 : Constant
  statusQA_c2 : Constant
  statusQA_c3 : Constant  Value=0
  statusQA_c4 : Constant  Value=3
  out_approvedSoup : Outport  PortName=approvedSoup  Element=batchId
  approvedSoup_el2 : Outport  PortName=approvedSoup  Element=volume_L
  approvedSoup_el3 : Outport  PortName=approvedSoup  Element=temp_C
  approvedSoup_el4 : Outport  PortName=approvedSoup  Element=contamination_ppm
  approvedSoup_el5 : Outport  PortName=approvedSoup  Element=flow_bps
  out_statusQA : Outport  Port=2  PortName=statusQA  Element=unitId
  statusQA_el2 : Outport  Port=2  PortName=statusQA  Element=opState
  statusQA_el3 : Outport  Port=2  PortName=statusQA  Element=faultCode
  statusQA_el4 : Outport  Port=2  PortName=statusQA  Element=power_kW
  statusQA_el5 : Outport  Port=2  PortName=statusQA  Element=health
  wires:
  statusQA_c3/1 -> statusQA_el3/1
  Gate_Fault_T_QC/1 -> En_Gate_Fault_T_QC/2, statusQA_el5/1
  statusQA_c2/1 -> statusQA_el2/1
  statusQA_c1/1 -> out_statusQA/1
  in_cookedSoup1/1 -> SoupSum/1
  statusQA_c4/1 -> statusQA_el4/1
  approvedSoup_c3/1 -> approvedSoup_el4/1
  approvedSoup_c1/1 -> out_approvedSoup/1
  in_cookedSoup2/1 -> SoupSum/2
  approvedSoup_c2/1 -> approvedSoup_el3/1
  Surge/3 -> Trm11/1
  in_directive/1 -> En_Gate_Fault_T_QC/1
  SoupSum/1 -> Surge/1
  QCDraw/1 -> Surge/2
  En_Gate_Fault_T_QC/1 -> QC/2
  QC/1 -> approvedSoup_el5/1, ToLitres/1
  Surge/1 -> QC/1
  Surge/2 -> Trm10/1
  QC/2 -> Trm8/1
  QC/3 -> Trm9/1
  QC/4 -> Trm12/1  "contamDetected_bps"
  QC/5 -> Trm13/1  "contamEscaped_bps"
  ToLitres/1 -> approvedSoup_el2/1

== system PhysicalLeanBroth/RefuelSkid ==
  in_directive : Inport  PortName=directive
  statusRefuel_c1 : Constant
  statusRefuel_c2 : Constant
  statusRefuel_c3 : Constant  Value=0
  statusRefuel_c4 : Constant  Value=8
  statusRefuel_h : Constant
  out_statusRefuel : Outport  PortName=statusRefuel  Element=unitId
  statusRefuel_el2 : Outport  PortName=statusRefuel  Element=opState
  statusRefuel_el3 : Outport  PortName=statusRefuel  Element=faultCode
  statusRefuel_el4 : Outport  PortName=statusRefuel  Element=power_kW
  statusRefuel_el5 : Outport  PortName=statusRefuel  Element=health
  wires:
  statusRefuel_h/1 -> statusRefuel_el5/1
  statusRefuel_c1/1 -> out_statusRefuel/1
  statusRefuel_c3/1 -> statusRefuel_el3/1
  statusRefuel_c4/1 -> statusRefuel_el4/1
  statusRefuel_c2/1 -> statusRefuel_el2/1

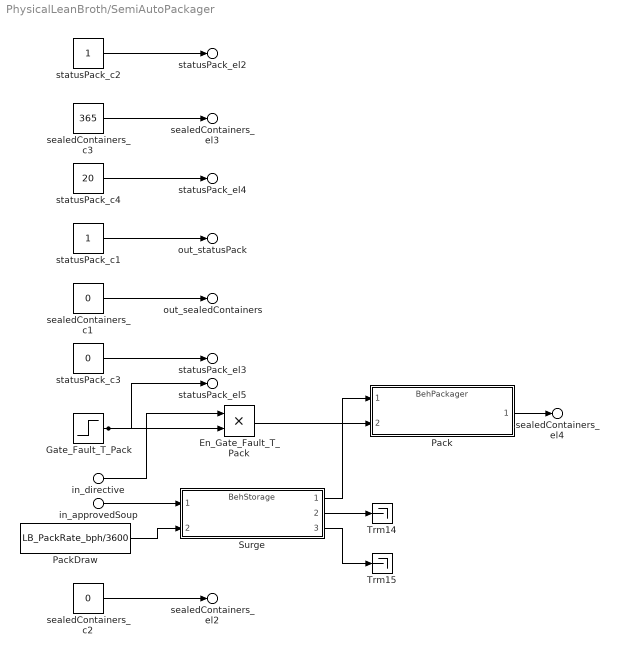
== system PhysicalLeanBroth/SemiAutoPackager ==
  in_approvedSoup : Inport  PortName=approvedSoup  Element=flow_bps
  in_directive : Inport  Port=2  PortName=directive  Element=setpoint
  En_Gate_Fault_T_Pack : Product
  Gate_Fault_T_Pack : Step  Time=Fault_T_Pack  InitialValue=1  FinalValue=0  SampleTime=0
  Pack : ModelReference  ModelNameDialog=BehPackager  UsingDefaultArgumentValue=0,0  SimulationMode=Normal  ModelReferenceVersion=1.4
  PackDraw : Constant  Value=LB_PackRate_bph/3600
  Surge : ModelReference  ModelNameDialog=BehStorage  UsingDefaultArgumentValue=0,0  SimulationMode=Normal  ModelReferenceVersion=1.3
  Trm14 : Terminator
  Trm15 : Terminator
  sealedContainers_c1 : Constant  Value=0
  sealedContainers_c2 : Constant  Value=0
  sealedContainers_c3 : Constant  Value=365
  statusPack_c1 : Constant
  statusPack_c2 : Constant
  statusPack_c3 : Constant  Value=0
  statusPack_c4 : Constant  Value=20
  out_sealedContainers : Outport  PortName=sealedContainers  Element=batchId
  sealedContainers_el2 : Outport  PortName=sealedContainers  Element=count
  sealedContainers_el3 : Outport  PortName=sealedContainers  Element=sealRating_days
  sealedContainers_el4 : Outport  PortName=sealedContainers  Element=flow_bps
  out_statusPack : Outport  Port=2  PortName=statusPack  Element=unitId
  statusPack_el2 : Outport  Port=2  PortName=statusPack  Element=opState
  statusPack_el3 : Outport  Port=2  PortName=statusPack  Element=faultCode
  statusPack_el4 : Outport  Port=2  PortName=statusPack  Element=power_kW
  statusPack_el5 : Outport  Port=2  PortName=statusPack  Element=health
  wires:
  statusPack_c2/1 -> statusPack_el2/1
  sealedContainers_c3/1 -> sealedContainers_el3/1
  statusPack_c4/1 -> statusPack_el4/1
  statusPack_c1/1 -> out_statusPack/1
  Gate_Fault_T_Pack/1 -> statusPack_el5/1, En_Gate_Fault_T_Pack/2
  sealedContainers_c1/1 -> out_sealedContainers/1
  statusPack_c3/1 -> statusPack_el3/1
  En_Gate_Fault_T_Pack/1 -> Pack/2
  in_directive/1 -> En_Gate_Fault_T_Pack/1
  in_approvedSoup/1 -> Surge/1
  PackDraw/1 -> Surge/2
  sealedContainers_c2/1 -> sealedContainers_el2/1
  Surge/1 -> Pack/1
  Surge/2 -> Trm14/1
  Surge/3 -> Trm15/1
  Pack/1 -> sealedContainers_el4/1

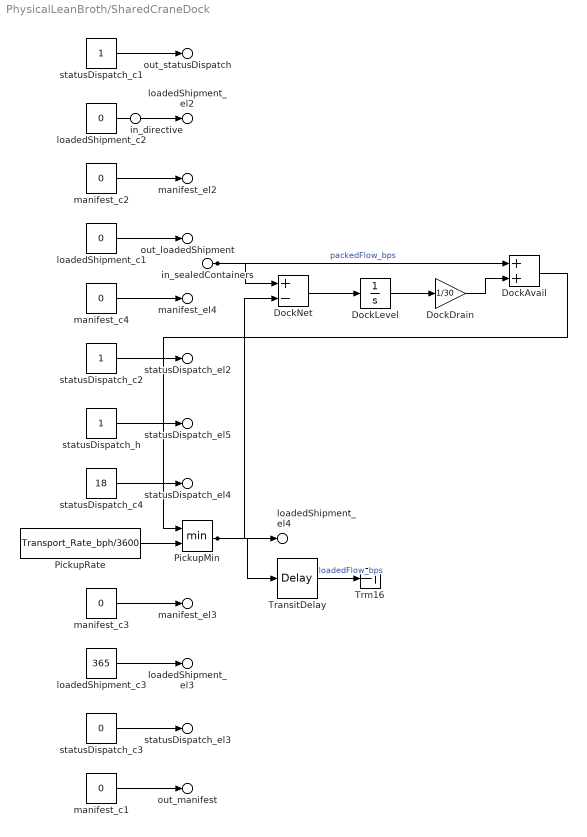
== system PhysicalLeanBroth/SharedCraneDock ==
  in_sealedContainers : Inport  PortName=sealedContainers  Element=flow_bps
  in_directive : Inport  Port=2  PortName=directive
  DockAvail : Sum
  DockDrain : Gain  Gain=1/30
  DockLevel : Integrator  LimitOutput=on  UpperSaturationLimit=600  LowerSaturationLimit=0
  DockNet : Sum  Inputs=+-
  PickupMin : MinMax  Inputs=2
  PickupRate : Constant  Value=Transport_Rate_bph/3600
  TransitDelay : TransportDelay  DelayTime=Transport_Latency_s
  Trm16 : Terminator
  loadedShipment_c1 : Constant  Value=0
  loadedShipment_c2 : Constant  Value=0
  loadedShipment_c3 : Constant  Value=365
  manifest_c{1..4} (4 alike) : Constant  Value=0
  statusDispatch_c1 : Constant
  statusDispatch_c2 : Constant
  statusDispatch_c3 : Constant  Value=0
  statusDispatch_c4 : Constant  Value=18
  statusDispatch_h : Constant
  out_loadedShipment : Outport  PortName=loadedShipment  Element=batchId
  loadedShipment_el2 : Outport  PortName=loadedShipment  Element=count
  loadedShipment_el3 : Outport  PortName=loadedShipment  Element=sealRating_days
  loadedShipment_el4 : Outport  PortName=loadedShipment  Element=flow_bps
  out_manifest : Outport  Port=2  PortName=manifest  Element=destinationId
  manifest_el2 : Outport  Port=2  PortName=manifest  Element=batchId
  manifest_el3 : Outport  Port=2  PortName=manifest  Element=count
  manifest_el4 : Outport  Port=2  PortName=manifest  Element=mass_kg
  out_statusDispatch : Outport  Port=3  PortName=statusDispatch  Element=unitId
  statusDispatch_el2 : Outport  Port=3  PortName=statusDispatch  Element=opState
  statusDispatch_el3 : Outport  Port=3  PortName=statusDispatch  Element=faultCode
  statusDispatch_el4 : Outport  Port=3  PortName=statusDispatch  Element=power_kW
  statusDispatch_el5 : Outport  Port=3  PortName=statusDispatch  Element=health
  wires:
  statusDispatch_c1/1 -> out_statusDispatch/1
  loadedShipment_c2/1 -> loadedShipment_el2/1
  loadedShipment_c1/1 -> out_loadedShipment/1
  manifest_c2/1 -> manifest_el2/1
  manifest_c4/1 -> manifest_el4/1
  statusDispatch_c4/1 -> statusDispatch_el4/1
  statusDispatch_c2/1 -> statusDispatch_el2/1
  statusDispatch_h/1 -> statusDispatch_el5/1
  in_sealedContainers/1 -> DockNet/1, DockAvail/1  "packedFlow_bps"
  PickupRate/1 -> PickupMin/2
  manifest_c3/1 -> manifest_el3/1
  loadedShipment_c3/1 -> loadedShipment_el3/1
  statusDispatch_c3/1 -> statusDispatch_el3/1
  manifest_c1/1 -> out_manifest/1
  PickupMin/1 -> DockNet/2, loadedShipment_el4/1, TransitDelay/1
  DockAvail/1 -> PickupMin/1
  DockNet/1 -> DockLevel/1
  TransitDelay/1 -> Trm16/1  "loadedFlow_bps"
  DockLevel/1 -> DockDrain/1
  DockDrain/1 -> DockAvail/2

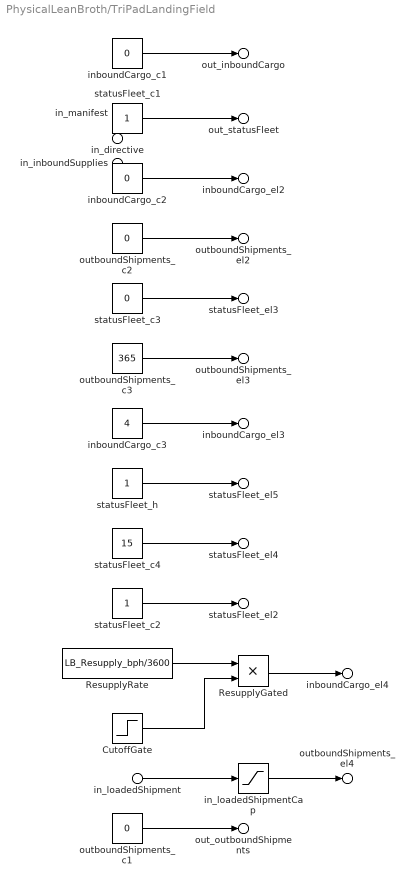
== system PhysicalLeanBroth/TriPadLandingField ==
  in_loadedShipment : Inport  PortName=loadedShipment  Element=flow_bps
  in_manifest : Inport  Port=2  PortName=manifest
  in_directive : Inport  Port=3  PortName=directive
  in_inboundSupplies : Inport  Port=4  PortName=inboundSupplies
  CutoffGate : Step  Time=Resupply_Cutoff_T  InitialValue=1  FinalValue=0  SampleTime=0
  ResupplyGated : Product
  ResupplyRate : Constant  Value=LB_Resupply_bph/3600
  in_loadedShipmentCap : Saturate  UpperLimit=0.0666666666667  LowerLimit=0
  inboundCargo_c1 : Constant  Value=0
  inboundCargo_c2 : Constant  Value=0
  inboundCargo_c3 : Constant  Value=4
  outboundShipments_c1 : Constant  Value=0
  outboundShipments_c2 : Constant  Value=0
  outboundShipments_c3 : Constant  Value=365
  statusFleet_c1 : Constant
  statusFleet_c2 : Constant
  statusFleet_c3 : Constant  Value=0
  statusFleet_c4 : Constant  Value=15
  statusFleet_h : Constant
  out_inboundCargo : Outport  PortName=inboundCargo  Element=palletId
  inboundCargo_el2 : Outport  PortName=inboundCargo  Element=mass_kg
  inboundCargo_el3 : Outport  PortName=inboundCargo  Element=temp_C
  inboundCargo_el4 : Outport  PortName=inboundCargo  Element=flow_bps
  out_outboundShipments : Outport  Port=2  PortName=outboundShipments  Element=batchId
  outboundShipments_el2 : Outport  Port=2  PortName=outboundShipments  Element=count
  outboundShipments_el3 : Outport  Port=2  PortName=outboundShipments  Element=sealRating_days
  outboundShipments_el4 : Outport  Port=2  PortName=outboundShipments  Element=flow_bps
  out_statusFleet : Outport  Port=3  PortName=statusFleet  Element=unitId
  statusFleet_el2 : Outport  Port=3  PortName=statusFleet  Element=opState
  statusFleet_el3 : Outport  Port=3  PortName=statusFleet  Element=faultCode
  statusFleet_el4 : Outport  Port=3  PortName=statusFleet  Element=power_kW
  statusFleet_el5 : Outport  Port=3  PortName=statusFleet  Element=health
  wires:
  inboundCargo_c1/1 -> out_inboundCargo/1
  ResupplyRate/1 -> ResupplyGated/1
  statusFleet_c1/1 -> out_statusFleet/1
  outboundShipments_c3/1 -> outboundShipments_el3/1
  inboundCargo_c2/1 -> inboundCargo_el2/1
  inboundCargo_c3/1 -> inboundCargo_el3/1
  outboundShipments_c2/1 -> outboundShipments_el2/1
  statusFleet_c3/1 -> statusFleet_el3/1
  statusFleet_h/1 -> statusFleet_el5/1
  statusFleet_c4/1 -> statusFleet_el4/1
  statusFleet_c2/1 -> statusFleet_el2/1
  CutoffGate/1 -> ResupplyGated/2
  in_loadedShipment/1 -> in_loadedShipmentCap/1
  outboundShipments_c1/1 -> out_outboundShipments/1
  ResupplyGated/1 -> inboundCargo_el4/1
  in_loadedShipmentCap/1 -> outboundShipments_el4/1
